simulink model "E5"  (R2014a)
settings: Solver=ode45  StartTime=0.0  StopTime=200  RelTol=1e-20
values from neighbouring files (symbols this model uses):
  s = tf('s')    [E5.m]
libraries: cstblocks x4, simulink x2
settings Model: Creator=Davide  LastModifiedBy=Davide

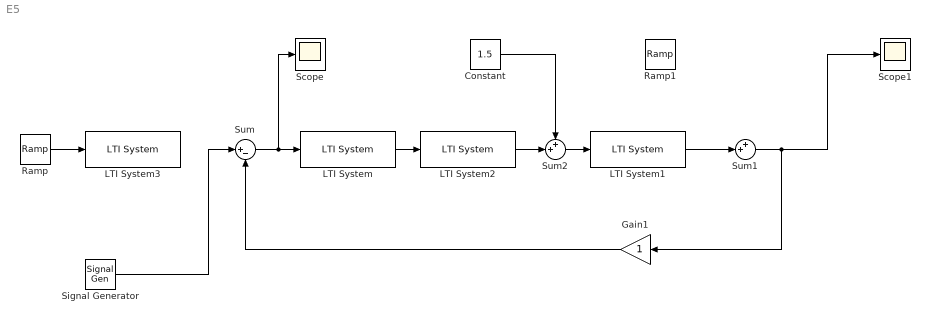
== system E5 ==
  Constant : Constant  Value=1.5
  Gain1 : Gain
  LTI System : cstblocks/LTI System  sys=C  IC=[]
  LTI System1 : cstblocks/LTI System  sys=F2  IC=[]
  LTI System2 : cstblocks/LTI System  sys=F1  IC=[]
  LTI System3 : cstblocks/LTI System  sys=1/s  IC=[]
  Ramp : simulink/Sources/Ramp  slope=1  start=0  X0=0
  Ramp1 : simulink/Sources/Ramp  slope=0.1  start=0  X0=0
  Scope : Scope
  Scope1 : Scope
  Signal Generator : SignalGenerator  Frequency=0.5  Units=rad/sec
  Sum : Sum  Inputs=|+-
  Sum1 : Sum  Inputs=++|
  Sum2 : Sum  Inputs=++|
  wires:
  Sum/1 -> Scope/1, LTI System/1
  LTI System/1 -> LTI System2/1
  Sum1/1 -> Gain1/1, Scope1/1
  LTI System2/1 -> Sum2/2
  LTI System1/1 -> Sum1/2
  Sum2/1 -> LTI System1/1
  Gain1/1 -> Sum/2
  Ramp/1 -> LTI System3/1
  Constant/1 -> Sum2/1
  Signal Generator/1 -> Sum/1
